simulink model "lab00"  (Simulink 5.0)
settings: Solver=ode45  StartTime=0.0  StopTime=10.0  RelTol=1e-3
settings Model: LastModifiedBy=Imed

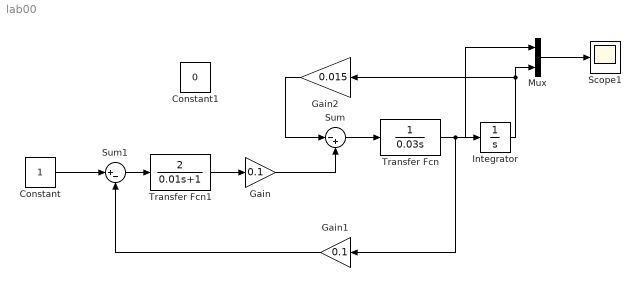
== system lab00 ==
  Constant : Constant
  Constant1 : Constant  Value=0
  Gain : Gain  Gain=0.1  SaturateOnIntegerOverflow=on
  Gain1 : Gain  Orientation=left  Gain=0.1  SaturateOnIntegerOverflow=on
  Gain2 : Gain  Orientation=left  Gain=0.015  SaturateOnIntegerOverflow=on
  Integrator : Integrator
  Mux : Mux  Inputs=2
  Scope1 : Scope
  Sum : Sum  Inputs=|-+  SaturateOnIntegerOverflow=on
  Sum1 : Sum  Inputs=|+-  SaturateOnIntegerOverflow=on
  Transfer Fcn : TransferFcn  Denominator=[0.03 0]
  Transfer Fcn1 : TransferFcn  Numerator=[2]  Denominator=[0.01 1]
  wires:
  Transfer Fcn/1 -> Integrator/1, Gain1/1, Mux/1
  Sum/1 -> Transfer Fcn/1
  Transfer Fcn1/1 -> Gain/1
  Gain/1 -> Sum/2
  Gain1/1 -> Sum1/2
  Sum1/1 -> Transfer Fcn1/1
  Constant/1 -> Sum1/1
  Mux/1 -> Scope1/1
  Gain2/1 -> Sum/1
  Integrator/1 -> Mux/2, Gain2/1
